simulink model "lab_5_qpsk_viterbi_sqrt"  (Simulink 8.0)
settings: Solver=VariableStepDiscrete  SolverMode=SingleTasking  StartTime=0.0  StopTime=inf  RelTol=1e-3
values from neighbouring files (symbols this model uses):
  EbNodB = EbNoVec(n)    [a1.m]    (also in a2.m = 11; cawgn.m = (1/4) * Nvar + 5; lab_5_Pber.m = 13; lab_5_Propyskna_Zdatnist.m = 11)
  Rb = Nvar    (= 24)    [lab_5_Propyskna_Zdatnist.m]    (also in lab_5_parameters.m = 14)
  Tb = 1/Rb    (= 0.0416666666667)    [lab_5_Propyskna_Zdatnist.m]    (also in lab_5_parameters.m = 0.0714285714286)
undefined symbols (not defined in the file or in its folder): figposition, Fs, sided, Two
libraries: commsink2 x6, commcnvcod2 x2, commdigbbndpm3 x2, dspsnks4 x2, commchan3 x1, commrandsrc2 x1, dspsigops x1, commfilt2 x1
CloseFcn:
  | clear convSigsOut
settings Model: RequirementInfo=9  Creator=mikem  LastModifiedBy=alex  CovMetricSettings=d  ExtModeTrigMode=oneshot  ExtModeArmWhenConnect=off
settings DataIOCC: LimitDataPoints=off  SignalLoggingSaveFormat=ModelDataLogs  SaveOutput=off  SaveTime=off  SignalLoggingName=convSigsOut
settings OptimizationCC: BlockReduction=off  BooleanDataType=off  InitFltsAndDblsToZero=on
settings DebuggingCC: SaveWithParameterizedLinksMsg=none  SignalResolutionControl=TryResolveAllWithWarning  SolverPrmCheckMsg=none  MultiTaskDSMMsg=warning  MultiTaskCondExecSysMsg=none  IntegerOverflowMsg=none  FcnCallInpInsideContextMsg=UseLocalSettings  StrictBusMsg=None
settings HardwareCC: TargetUnknown=on
settings RTWCC: IncludeERTFirstTime=on
settings GRTTargetCC: TargetFcnLib=ansi_tfl_tmw.mat  CombineOutputUpdateFcns=off  GRTInterface=on

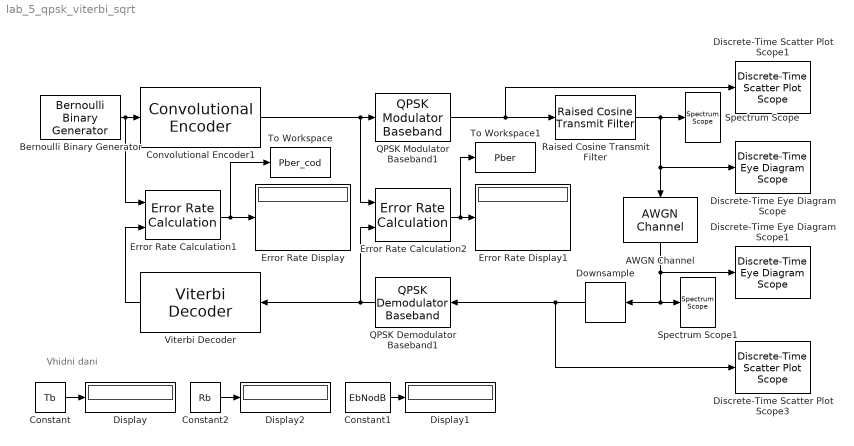
== system lab_5_qpsk_viterbi_sqrt ==
  note: Vhidni dani
  AWGN Channel : commchan3/AWGN Channel  InputProcessing=Inherited (this choice will be removed - see release notes)  seed=54321  noiseMode="Signal to noise ratio  (Es/No)"  EbNodB=5  EsNodB=EbNodB+10*log10(1/2)  SNRdB=5  bitsPerSym=2  Ps=1  Tsym=1/8*Tb  variance=1
  Bernoulli Binary Generator : commrandsrc2/Bernoulli Binary Generator  P=0.5  seed=12345  Ts=Tb  frameBased=on  sampPerFrame=1  orient=off  outDataType=double
  Constant : Constant  Value=Tb
  Constant1 : Constant  Value=EbNodB
  Constant2 : Constant  Value=Rb
  Convolutional Encoder1 : commcnvcod2/Convolutional Encoder  trellis=poly2trellis(7, [171 133])  opMode=Continuous  DelayedResetAction=off  hasIniStPort=off  hasFinStPort=off  usePuncVector=off  punctureVector=[1; 1; 0; 1; 0; 1]  reset=Unused parameter value
  Discrete-Time Eye Diagram Scope : commsink2/Discrete-Time Eye Diagram Scope  Tag=EyeDiagram  sampPerSymb=8  offsetEye=0  symbPerTrace=2  numTraces=10  numNewFrames=1  LineStyles=-  LineColors=b  dupPoints=on  fading=on  render=on  AxisGrid=on  yMin=-1.14712819935187  yMax=1.15234241843983  inphaseLabel=In-phase Amplitude  quadratureLabel=Quadrature Amplitude  openScopeAtSimStart=off  dispDiagram=In-phase and Quadrature  FrameNumber=off  FigPos=[360 54 560 644]  figTitle=Eye Diagram  block_type_=eye  numLinesMax=8
  Discrete-Time Eye Diagram Scope1 : commsink2/Discrete-Time Eye Diagram Scope  Tag=EyeDiagram  sampPerSymb=8  offsetEye=0  symbPerTrace=2  numTraces=100  numNewFrames=1  LineStyles=-  LineColors=b  dupPoints=on  fading=on  render=on  AxisGrid=on  yMin=-1.5  yMax=1.5  inphaseLabel=In-phase Amplitude  quadratureLabel=Quadrature Amplitude  openScopeAtSimStart=off  dispDiagram=In-phase and Quadrature  FrameNumber=off  FigPos=[360 54 560 644]  figTitle=Eye Diagram  block_type_=eye  numLinesMax=8
  Discrete-Time Scatter Plot Scope1 : commsink2/Discrete-Time Scatter Plot Scope  Tag=ScatterPlot  sampPerSymb=1  offsetEye=0  numTraces=40  numNewFrames=10  LineMarkers=.  LineColors=b  fading=on  render=on  AxisGrid=on  xMin=-0.777817459305202  xMax=0.781352993211135  yMin=-0.0724784450716212  yMax=1.48669200744472  inphaseLabel=In-phase Amplitude  quadratureLabel=Quadrature Amplitude  openScopeAtSimStart=on  FrameNumber=off  FigPos=[360 138 560 560]  figTitle=Scatter Plot  numLinesMax=8  block_type_=scatter
  Discrete-Time Scatter Plot Scope3 : commsink2/Discrete-Time Scatter Plot Scope  Tag=ScatterPlot  sampPerSymb=1  offsetEye=0  numTraces=40  numNewFrames=10  LineMarkers=.  LineColors=b  fading=on  render=on  AxisGrid=on  xMin=-1.5  xMax=1.5  yMin=-1.5  yMax=1.5  inphaseLabel=In-phase Amplitude  quadratureLabel=Quadrature Amplitude  openScopeAtSimStart=on  FrameNumber=off  FigPos=[360 138 560 560]  figTitle=Scatter Plot  numLinesMax=8  block_type_=scatter
  Display : Display
  Display1 : Display
  Display2 : Display
  Downsample : dspsigops/Downsample  N=8  phase=0  InputProcessing=Inherited (this choice will be removed - see release notes)  RateOptions=Enforce single-rate processing  smode=Allow multirate  fmode=Maintain input frame rate  ic=0
  Error Rate Calculation1 : commsink2/Error Rate Calculation  N=3/1*1+96  st_delay=0  cp_mode=Entire frame  subframe=[]  PMode=Port  WsName=ErrorVec  RsMode2=off  stop=off  numErr=100  maxBits=1e7
  Error Rate Calculation2 : commsink2/Error Rate Calculation  N=3/1*2  st_delay=0  cp_mode=Entire frame  subframe=[]  PMode=Port  WsName=ErrorVec  RsMode2=off  stop=off  numErr=100  maxBits=1e6
  Error Rate Display : Display
  Error Rate Display1 : Display
  QPSK Demodulator Baseband1 : commdigbbndpm3/QPSK Demodulator Baseband  Ph=pi/4  Dec=Gray  OutType=Integer  DecType=Hard decision  VarSource=Dialog  Variance=1  outDtype1=Inherit via internal rule  outDtype2=Inherit via internal rule  derotateFactorWordLen=16
  QPSK Modulator Baseband1 : commdigbbndpm3/QPSK Modulator Baseband  InType=Integer  Enc=Gray  Ph=pi/4  outDtype=double  outWordLen=16  outUDDataType=sfix(16)  outFracLenMode=Best precision  outFracLen=15
  Raised Cosine Transmit Filter : commfilt2/Raised Cosine Transmit Filter  filtType=Normal  D=3  R=0.5  sampMode=Mute  saveAsFlag=0  N=8  framing=Maintain input frame rate  InputProcessing=Columns as channels (frame based)  checkGain=Normalized  filterGain=1  checkCoeff=off  variableName=rcTxFilt  launchFVT=off  roundingMode=Floor  overflowMode=off
      link override Check Signal Attributes: Frame=Frame-based  Dimensions=Column vector (2-D) or scalar
      link override FIR Interpolation: framing=Maintain input frame rate
  Spectrum Scope : dspsnks4/Spectrum Scope  ScopeProperties=on  Domain=Frequency  HorizSpan=1  UseBuffer=on  BufferSize=256  Overlap=0  TreatMby1Signals=M channels  inpFftLenInherit=off  FFTlength=128  numAvg=20  DisplayProperties=off  AxisGrid=on  Memory=off  FrameNumber=off  AxisLegend=off  AxisZoom=off  OpenScopeAtSimStart=on  OpenScopeImmediately=off  FigPos="figposition([7    12    39    27])"  AxisProperties=off  XUnits=Hertz  XRange=Two-sided ((-Fs/2...Fs/2])  XDisplay=0  InheritXIncr=on  XIncr=1.0  XLabel=Samples  XLimit=Auto  YUnits=dBW/Hertz  XMax=1  XMin=0  YLabel=Magnitude-squared, dB  LineProperties=off  LineColors=[1 0 0]  wintypeSpecScope=Hann  RsSpecScope=50  betaSpecScope=5  winsampSpecScope=Periodic  XAxisParamsVer=6.8  isFrameUpgraded=on
      settings: YMin=-50  YMax=10
  Spectrum Scope1 : dspsnks4/Spectrum Scope  ScopeProperties=on  Domain=Frequency  HorizSpan=1  UseBuffer=on  BufferSize=256  Overlap=0  TreatMby1Signals=M channels  inpFftLenInherit=off  FFTlength=128  numAvg=20  DisplayProperties=off  AxisGrid=on  Memory=off  FrameNumber=off  AxisLegend=off  AxisZoom=off  OpenScopeAtSimStart=on  OpenScopeImmediately=off  FigPos="figposition([49    12    39    27])"  AxisProperties=off  XUnits=Hertz  XRange=Two-sided ((-Fs/2...Fs/2])  XDisplay=0  InheritXIncr=on  XIncr=1.0  XLabel=Samples  XLimit=Auto  YUnits=dBW/Hertz  XMax=1  XMin=0  YLabel=Magnitude-squared, dB  LineProperties=off  LineColors=[1 0 0]  wintypeSpecScope=Hann  RsSpecScope=50  betaSpecScope=5  winsampSpecScope=Periodic  XAxisParamsVer=6.8  isFrameUpgraded=on
      settings: YMin=-10  YMax=10
  To Workspace : ToWorkspace  VariableName=Pber_cod  SampleTime=-1
      settings: MaxDataPoints=1
  To Workspace1 : ToWorkspace  VariableName=Pber  SampleTime=-1
      settings: MaxDataPoints=1
  Viterbi Decoder : commcnvcod2/Viterbi Decoder  trellis=poly2trellis(7, [171 133])  isPunctured=off  punctureVector=[1; 1; 0; 1; 0; 1]  erasures=off  dectype=Hard decision  runSigValErrCheck=off  nsdecb=4  smWordLength=16  tbdepth=96  opmode=Continuous  reset=off  outDataType=double  delayedResetAction=off
  wires:
  Convolutional Encoder1/1 -> QPSK Modulator Baseband1/1, Error Rate Calculation2/1
  Viterbi Decoder/1 -> Error Rate Calculation1/2
  QPSK Modulator Baseband1/1 -> Raised Cosine Transmit Filter/1, Discrete-Time Scatter Plot Scope1/1
  Raised Cosine Transmit Filter/1 -> AWGN Channel/1, Discrete-Time Eye Diagram Scope/1, Spectrum Scope/1
  QPSK Demodulator Baseband1/1 -> Viterbi Decoder/1, Error Rate Calculation2/2
  Bernoulli Binary Generator/1 -> Convolutional Encoder1/1, Error Rate Calculation1/1
  AWGN Channel/1 -> Downsample/1, Spectrum Scope1/1, Discrete-Time Eye Diagram Scope1/1
  Downsample/1 -> QPSK Demodulator Baseband1/1, Discrete-Time Scatter Plot Scope3/1
  Error Rate Calculation1/1 -> Error Rate Display/1, To Workspace/1
  Error Rate Calculation2/1 -> Error Rate Display1/1, To Workspace1/1
  Constant/1 -> Display/1
  Constant1/1 -> Display1/1
  Constant2/1 -> Display2/1
